simulink model "nms_3Dmodel"  (Simulink 8.5)
settings: Solver=ode15s  StartTime=0.0  StopTime=30  FixedStep=1e-3  RelTol=1e-3  AbsTol=1e-4
InitFcn:
  | runScripts;
values from neighbouring files (symbols this model uses):
  ankle_height = 0.08    [nms_MechInit.m]
  c = 0.05    [nms_MechInit.m]
  c_jointstop = 0.3 / (pi/180)    (= 17.1887338539)    [nms_MechInit.m]
  CtrlPar_FP = [alpha0 alpha_cd alpha_cv]    [setCtrlPar.m]
  CtrlPar_FP_R = [R_hipR0 R_hipR_cd R_hipR_cv]    [setCtrlPar.m]
  CtrlPar_LL = l_clr    [setCtrlPar.m]
  CtrlPar_St = [StPreStim St_M1 St_M2 St_M3 St_M4 St_M5]    [setCtrlPar.m]
  CtrlPar_St_R = [R_StPreStim R_St_M1 R_St_M3 R_St_M4]    [setCtrlPar.m]
  CtrlPar_Sw = [SwPreStim SwPhasePari SwPhaseParii SwCtrlPar_H SwCtrlPar_A      SwCtrlPar_Ki SwCtrlPar_Kii SwCtrlPar_Kiii SwCtrlPar_StP]    [setCtrlPar.m]
  CtrlPar_Sw_R = [R_SwPreStim R_Sw_M6]    [setCtrlPar.m]
  CtrlPar_theta0 = parBlCtrl(1)      *1*pi/180    [setCtrlPar.m]
  CtrlPar_Tr = [Tr_St_sup Tr_Sw]    [setCtrlPar.m]
  CtrlPar_Tr_R = [R_Tr_St_sup R_Tr_Sw]    [setCtrlPar.m]
  D12_F = 0.16    [nms_MechInit.m]
  D12_S = D12_S - ankle_height/2    (= 0.46)    [nms_MechInit.m]
  D12_T = D12_T - ankle_height/2    (= 0.46)    [nms_MechInit.m]
  D12z_T = 0.1    [nms_MechInit.m]
  D13_F = 0.20    (= 0.2)    [nms_MechInit.m]
  D1G_F = 0.14    [nms_MechInit.m]
  D1G_HAT = 0.35    [nms_MechInit.m]
  D1G_S = D1G_S - ankle_height/4    (= 0.28)    [nms_MechInit.m]
  D1G_T = D1G_T - ankle_height/4    (= 0.28)    [nms_MechInit.m]
  D1Gy_F = ankle_height*D1G_F/D12_F    (= 0.07)    [nms_MechInit.m]
  d_fBall = 0.1    [nms_MechInit.m]
  d_fHeel = 0.05    [nms_MechInit.m]
  DeltaThRef = 5e-3    (= 0.005)    [nms_MechInit.m]
  eref = 0.04    [nms_MechInit.m]
  FmaxBFSH = 350    [nms_MechInit.m]
  FmaxGAS = 1500    [nms_MechInit.m]
  FmaxGLU = 1500    [nms_MechInit.m]
  FmaxHAB = 3000    [nms_MechInit.m]
  FmaxHAD = 4500    [nms_MechInit.m]
  FmaxHAM = 3000    [nms_MechInit.m]
  FmaxHFL = 2000    [nms_MechInit.m]
  FmaxRF = 1200    [nms_MechInit.m]
  FmaxSOL = 4000    [nms_MechInit.m]
  FmaxTA = 800    [nms_MechInit.m]
  FmaxVAS = 6000    [nms_MechInit.m]
  In_F = 0.005    [nms_MechInit.m]
  In_HAT = 2.5    [nms_MechInit.m]
  In_S = 0.05    [nms_MechInit.m]
  In_T = 0.15    [nms_MechInit.m]
  init_a_tgt = 70*pi/180    (= 1.2217304764)    [setInitPar.m]
  init_a_tgtR = 90*pi/180    (= 1.57079632679)    [setInitPar.m]
  Inx_F = 0.0007    [nms_MechInit.m]
  Inx_HAT = 1.0    (= 1)    [nms_MechInit.m]
  Inx_S = 0.003    [nms_MechInit.m]
  Inx_T = 0.03    [nms_MechInit.m]
  Iny_F = 0.005    [nms_MechInit.m]
  Iny_HAT = 4.0    (= 4)    [nms_MechInit.m]
  Iny_S = 0.05    [nms_MechInit.m]
  Iny_T = 0.15    [nms_MechInit.m]
  K = 5    [nms_MechInit.m]
  k_gn = k_gn/2    (= 39240)    [nms_MechInit.m]
  k_gt = k_gt/2    (= 3924)    [nms_MechInit.m]
  k_pressure = m_HAT * 9.81 / DeltaThRef    (= 104967)    [nms_MechInit.m]
  leg_l = [D12_T D12_S]    [nms_MechInit.m]
  LongDelay = 0.020/2    (= 0.01)    [nms_MechInit.m]
  LongLoopDelay = 0.030    (= 0.03)    [nms_MechInit.m]
  loptBFSH = 0.12    [nms_MechInit.m]
  loptGAS = 0.05    [nms_MechInit.m]
  loptGLU = 0.11    [nms_MechInit.m]
  loptHAB = 0.09    [nms_MechInit.m]
  loptHAD = 0.10    (= 0.1)    [nms_MechInit.m]
  loptHAM = 0.10    (= 0.1)    [nms_MechInit.m]
  loptHFL = 0.11    [nms_MechInit.m]
  loptRF = 0.08    [nms_MechInit.m]
  loptSOL = 0.04    [nms_MechInit.m]
  loptTA = 0.06    [nms_MechInit.m]
  loptVAS = 0.08    [nms_MechInit.m]
  lslackBFSH = 0.10    (= 0.1)    [nms_MechInit.m]
  lslackGAS = 0.40    (= 0.4)    [nms_MechInit.m]
  lslackGLU = 0.13    [nms_MechInit.m]
  lslackHAB = 0.07    [nms_MechInit.m]
  lslackHAD = 0.18    [nms_MechInit.m]
  lslackHAM = 0.31    [nms_MechInit.m]
  lslackHFL = 0.10    (= 0.1)    [nms_MechInit.m]
  lslackRF = 0.35    [nms_MechInit.m]
  lslackSOL = 0.26    [nms_MechInit.m]
  lslackTA = 0.24    [nms_MechInit.m]
  lslackVAS = 0.23    [nms_MechInit.m]
  m_F = 1.25    [nms_MechInit.m]
  m_HAT = 53.5    [nms_MechInit.m]
  m_S = 3.5    [nms_MechInit.m]
  m_T = 8.5    [nms_MechInit.m]
  MidDelay = 0.010/2    (= 0.005)    [nms_MechInit.m]
  mu_slide = 0.8    [nms_MechInit.m]
  mu_stick = 0.9    [nms_MechInit.m]
  N = 1.5    [nms_MechInit.m]
  phi12_LowLimit = 70*pi/180    (= 1.2217304764)    [nms_MechInit.m]
  phi12_UpLimit = 130*pi/180    (= 2.26892802759)    [nms_MechInit.m]
  phi23_UpLimit = 175*pi/180    (= 3.05432619099)    [nms_MechInit.m]
  phi34_UpLimit = 230*pi/180    (= 4.01425727959)    [nms_MechInit.m]
  phi34R_LowLimit = -15*pi/180    (= -0.261799387799)    [nms_MechInit.m]
  phi34R_UpLimit = 50*pi/180    (= 0.872664625997)    [nms_MechInit.m]
  phimaxGASa = 100*pi/180    (= 1.74532925199)    [nms_MechInit.m]
  phimaxGASk = 140*pi/180    (= 2.44346095279)    [nms_MechInit.m]
  phimaxRFk = 165*pi/180    (= 2.87979326579)    [nms_MechInit.m]
  phimaxSOL = 100*pi/180    (= 1.74532925199)    [nms_MechInit.m]
  phimaxTA = 80*pi/180    (= 1.3962634016)    [nms_MechInit.m]
  phimaxVAS = 165*pi/180    (= 2.87979326579)    [nms_MechInit.m]
  phirefBFSH = 160*pi/180    (= 2.79252680319)    [nms_MechInit.m]
  phirefGASa = 80*pi/180    (= 1.3962634016)    [nms_MechInit.m]
  phirefGASk = 165*pi/180    (= 2.87979326579)    [nms_MechInit.m]
  phirefGLU = 120*pi/180    (= 2.09439510239)    [nms_MechInit.m]
  phirefHAB = 10*pi/180    (= 0.174532925199)    [nms_MechInit.m]
  phirefHAD = 15*pi/180    (= 0.261799387799)    [nms_MechInit.m]
  phirefHAMh = 150*pi/180    (= 2.61799387799)    [nms_MechInit.m]
  phirefHAMk = 180*pi/180    (= 3.14159265359)    [nms_MechInit.m]
  phirefHFL = 160*pi/180    (= 2.79252680319)    [nms_MechInit.m]
  phirefRFh = 170*pi/180    (= 2.96705972839)    [nms_MechInit.m]
  phirefRFk = 125*pi/180    (= 2.18166156499)    [nms_MechInit.m]
  phirefSOL = 90*pi/180    (= 1.57079632679)    [nms_MechInit.m]
  phirefTA = 110*pi/180    (= 1.91986217719)    [nms_MechInit.m]
  phirefVAS = 120*pi/180    (= 2.09439510239)    [nms_MechInit.m]
  phiScaleGASa = acos(rGASamin/rGASamax)/(phiminGASa-phimaxGASa)    [nms_MechInit.m]
  phiScaleGASk = acos(rGASkmin/rGASkmax)/(phiminGASk-phimaxGASk)    [nms_MechInit.m]
  phiScaleRFk = acos(rRFkmin/rRFkmax)/(phiminRFk-phimaxRFk)    [nms_MechInit.m]
  phiScaleSOL = acos(rSOLmin/rSOLmax)/(phiminSOL-phimaxSOL)    [nms_MechInit.m]
  phiScaleTA = acos(rTAmin/rTAmax)/(phiminTA-phimaxTA)    [nms_MechInit.m]
  ... (+74 more)
undefined symbols (not defined in the file or in its folder): magnitude, sgn
libraries: mblibv1 x88, simulink x44, simulink_extras x38
(part 1 of 14)
settings Model: Creator=hgeyer  LastModifiedBy=smsong
settings SolverCC: ZeroCrossAlgorithm=Adaptive
settings DataIOCC: LimitDataPoints=off  SignalLogging=off
settings OptimizationCC: BooleanDataType=off  InitFltsAndDblsToZero=on
settings DebuggingCC: SaveWithParameterizedLinksMsg=none  SignalResolutionControl=TryResolveAllWithWarning  MaxConsecutiveZCsMsg=warning  SolverPrmCheckMsg=warning  MultiTaskDSMMsg=warning  MultiTaskCondExecSysMsg=none  FcnCallInpInsideContextMsg=UseLocalSettings  UnconnectedLineMsg=none
settings GRTTargetCC: TargetFcnLib=ansi_tfl_tmw.mat
settings SimMechanicsCC: VisOnUpdateDiagram=on  VisDuringSimulation=on  VisSampleTime=0.01  HighlightModel=off  AutoFitVis=GROWTOFIT  LastVizWinPosition=[126 112 1245 592]  CamPosition=[10.9406;3.67889;8.45305;]  CamTarget=[0.97968;0.591012;-0.112655;]  CamUpVector=[-0.166765;0.973419;-0.156985;]  CamHeight=3.15748  VisBackgroundColor=[0.9;0.9;0.95;]  DefaultBodyColor=[1;0;0;]
settings ConfigurationSet: Description=SimMechanics 2G

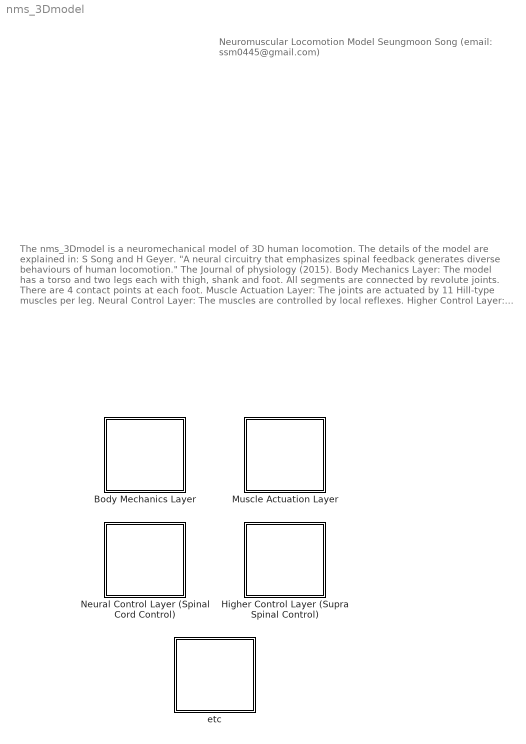
== system nms_3Dmodel ==
  note: Neuromuscular Locomotion Model
      | Seungmoon Song
      | (email: ssm0445@gmail.com)
  note: The nms_3Dmodel is a neuromechanical model of 3D human locomotion.
      | The details of the model are explained in:
      | S Song and H Geyer. "A neural circuitry that emphasizes spinal feedback
      | generates diverse behaviours of human locomotion." The Journal of physiology (2015).
      |
      | Body Mechanics Layer:
      | The model has a torso and two legs each with thigh, shank and foot.
      | All segments are connected by revolute joints.
      | There are 4 contact points at each foot.
      |
      | Muscle Actuation Layer:
      | The joints are actuated by 11 Hill-type muscles per leg.
      |
      | Neural Control Layer:
      | The muscles are controlled by local reflexes.
      |
      | Higher Control Layer:
      | The reflex pathways are modulated by the higher layer control.
  Body Mechanics Layer : Subsystem
  Higher Control Layer (Supra Spinal Control) : Subsystem
  Muscle Actuation Layer : Subsystem
  Neural Control Layer (Spinal Cord Control) : Subsystem
  etc : Subsystem
